simulink model "Ex310"  (R2021b)
settings: Solver=VariableStepAuto  StartTime=0.0  StopTime=10.0  RelTol=1e-3
settings Model: Creator=abdul  LastModifiedBy=abdul

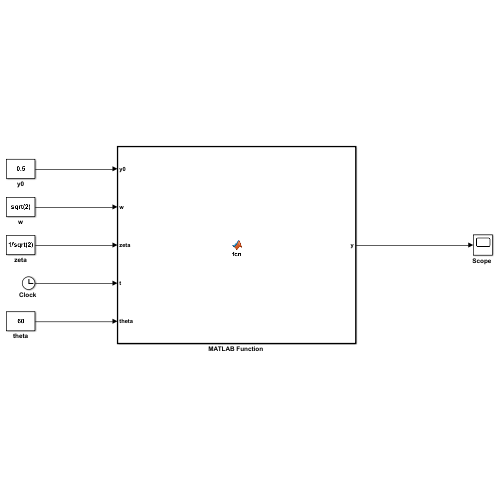
[thumbnail: Simulink's stored preview of the top-level diagram]
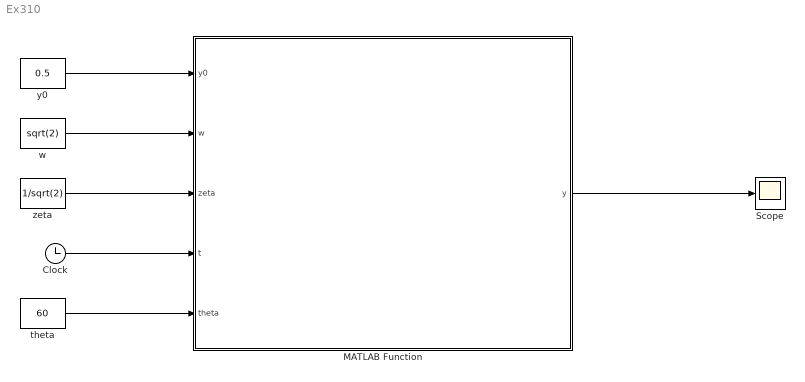
== system Ex310 ==
  "Clock " : Clock
  "MATLAB Function " : MATLAB Function  TreatAsAtomicUnit=on
  "Scope " : Scope
  theta : Constant  Value=60
  w : Constant  Value=sqrt(2)
  y0 : Constant  Value=0.5
  zeta : Constant  Value=1/sqrt(2)
  wires:
  "Clock "/1 -> "MATLAB Function "/4(t)
  y0/1 -> "MATLAB Function "/1(y0)
  theta/1 -> "MATLAB Function "/5(theta)
  zeta/1 -> "MATLAB Function "/3(zeta)
  w/1 -> "MATLAB Function "/2(w)
  "MATLAB Function "/1(y) -> "Scope "/1

== matlab function Ex310/MATLAB Function  ==
  data: y0 input; y output; w input; zeta input; t input; theta input
function y = fcn(y0,w,zeta,t,theta)
y=(y0/sqrt(1-zeta*zeta))*exp(-zeta*w*t)*sin(w*sqrt(1-zeta*zeta)*t+theta*pi/180);
end
